simulink model "downsample_ref3"  (Simulink 4.00)
settings: Solver=FixedStepDiscrete  SolverMode=MultiTasking  StartTime=0.0  StopTime=30  RelTol=1e-3
PostLoadFcn:
  | set_param(gcs,'SimulationCommand','Update')
libraries: dspsigops x1, dspsrcs3 x1
settings Model: RequirementInfo=9  LastModifiedBy=dfass  LimitDataPoints=off  ExtModeTrigMode=oneshot  ExtModeArmWhenConnect=off  BlockReductionOpt=off

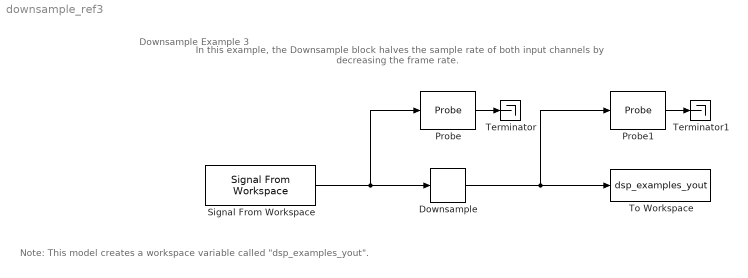
== system downsample_ref3 ==
  note: Downsample Example 3
  note: In this example, the Downsample block halves the sample rate
      | of both input channels by decreasing the frame rate.
  note: Note: This model creates a workspace variable called "dsp_examples_yout".
  Downsample : dspsigops/Downsample  N=2  phase=1  ic=[11 -11;12 -12;13 -13;14 -14]  smode=Allow multirate  fmode=Maintain input frame size
  Probe : Probe  ProbeWidth=off  ProbeSampleTime=on  ProbeComplexSignal=off  ProbeSignalDimensions=off
  Probe1 : Probe  ProbeWidth=off  ProbeSampleTime=on  ProbeComplexSignal=off  ProbeSignalDimensions=off
  Signal From Workspace : dspsrcs3/Signal From Workspace  X=[(1:100)' (-1:-1:-100)']  Ts=0.25  nsamps=4  OutputAfterFinalValue=Setting To Zero
  Terminator : Terminator
  Terminator1 : Terminator
  To Workspace : ToWorkspace  VariableName=dsp_examples_yout  SampleTime=-1  SaveFormat=Array
  wires:
  Downsample/1 -> To Workspace/1, Probe1/1
  Signal From Workspace/1 -> Probe/1, Downsample/1
  Probe/1 -> Terminator/1
  Probe1/1 -> Terminator1/1
